simulink model "mavros_simulink_test"  (R2024b)
settings: Solver=FixedStepAuto  StartTime=0.0  StopTime=inf  FixedStep=0.01  RelTol=1e-3
undefined symbols (not defined in the file): altitude, coordinate_frame, custom_mode, custom_mode_SL_Info, latitude, longitude, min_pitch, position, start_index, type_mask, waypoints, waypoints_SL_Info, yaw
libraries: ros2lib x14, simulink_extras x1, robotcorelib x1, aerolibconvert2 x1
settings Model: Creator=hiro  LastModifiedBy=hiro

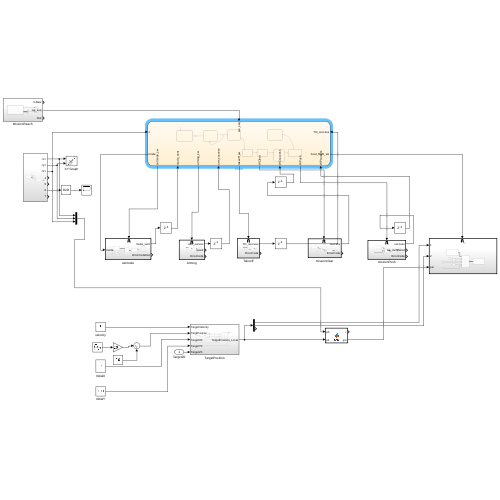
[thumbnail: Simulink's stored preview of the top-level diagram]
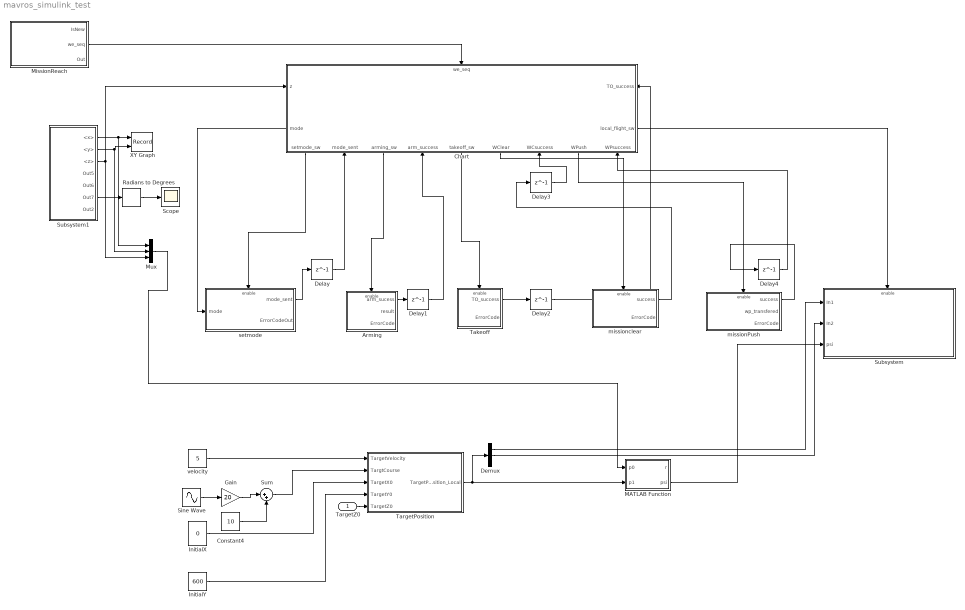
== system mavros_simulink_test ==
  TargetZ0 : Inport
  Arming : Subsystem
  Chart : Stateflow chart  TreatAsAtomicUnit=on
      settings: PortSchema="{\"entries\":[{\"content\":{\"sides\":[{\"content\":{\"connectorIds\":[\"In2\",\"Out1\"]},\"type\":\"ConnectorPlacement.EquallySpacedRectSide\",\"uuid\":\"83bdd756-f1da-4c0c-8304-adf84ef4ab4e\"},{\"content\":{\"connectorIds\":[\"In3\",\"Out2\"],\"side\":\"RIGHT\"},\"type\":\"ConnectorPlacement.EquallySpacedRectSide\",\"uuid\":\"a37bf1db-0ec9-4e4d-8590-be40530fb588\"},{\"content\":{\"connectorIds\":[\"In1\"],\"side\":\"TOP\"},\"type\":\"ConnectorPlacement.EquallySpacedRectSide\",\"uuid\":\"a8adb6fc-024d-410d-a7f4-a90207d0e0c2\"},{\"content\":{\"connectorIds\":[\"Out3\",\"In6\",\"Out4\",\"In7\",\"Out5\",\"Out6\",\"In4\",\"Out7\",\"In5\"],\"side\":\"BOTTOM\"},\"type\":\"ConnectorPlacement.EquallySpacedRectSide\",\"uuid\":\"fe5d25e7-d449-445c-b7fc-97e28e307bb9\"}]},\"type\":\"ConnectorPlacement.EquallySpacedConnector\",\"uuid\":\"da6e0aaf-ad56-47fd-8214-9fe2a8d7ed6f\"}],\"packageUris\":[\"http://schema.mathworks.com/mf0/Connector/R2020b\"],\"version\":\"1.0\"}"
  Constant4 : Constant  Value=10  SampleTime=0
  Delay{,1..4} (5 alike) : Delay  DelayLength=1  InitialCondition=0
  Demux : Demux  Outputs=3
  Gain : Gain  Gain=20
  InitialX : Constant  Value=0
  InitialY : Constant  Value=600
  MATLAB Function : MATLAB Function  TreatAsAtomicUnit=on
  MissionReach : Subsystem
  Mux : Mux  Inputs=3
  Radians to Degrees : simulink_extras/Transformations/Radians to Degrees
  Scope : Scope
  Sine Wave : Sin  Frequency=0.1  SampleTime=0
  Subsystem : Subsystem
  Subsystem1 : Subsystem
  Sum : Sum  Inputs=|++
  Takeoff : Subsystem
  TargetPosition : Subsystem
  XY Graph : Record  FileSettingsInternal="{\"entries\":[{\"content\":{\"excelSettings\":{\"content\":{},\"type\":\"Streamout.ExcelSettings\"}},\"type\":\"Streamout.FileSettingStorage\",\"uuid\":\"\"}],\"packageUris\":[\"http:\\/\\/schema.mathworks.com\\/mf0\\/streamout_blocks\\/R2020a\"],\"version\":\"1.0\"}"  Layout=[1 1]  SignalsInternal="{\"entries\":[{\"content\":{\"signals\":[{\"content\":{\"blockPath\":[],\"dimensions\":[1],\"domain\":\"\",\"lineColor\":\"#a2142f\",\"plots\":[ 1 ],\"port\":1,\"sid\":[\"\"],\"signalID\":1,\"signalName\":\"Subsystem1:1\"},\"type\":\"RecordBlkView.Signal\",\"uuid\":\"\"},{\"content\":{\"blockPath\":[],\"dimensions\":[1],\"domain\":\"\",\"lineColor\":\"#139fff\",\"plots\":[ 1 ],\"port\":2,\"sid\":[\"\"],\"signalID\":2,\"signalName\":\"Subsystem1:2\"},\"type\":\"RecordBlkView.Signal\",\"uuid\":\"\"}]},\"type\":\"RecordBlkView.InputSignals\",\"uuid\":\"\"}],\"packageUris\":[\"http:\\/\\/schema.mathworks.com\\/mf0\\/streamout_blocks\\/R2020a\"],\"version\":\"1.0\"}"  VisualizationBindings="{\"xyplotplugin\":{\"info\":[{\"series\":[{\"bindingParametersList\":[{\"parameter\":\"X-Axis\",\"signalID\":1,\"signalName\":\"Subsystem1:1\"},{\"parameter\":\"Y-Axis\",\"signalID\":2,\"signalName\":\"Subsystem1:2\"}],\"seriesID\":0}],\"subplotID\":1}]}}"  CompatibilityTag=XY
  missionPush : Subsystem
  missionclear : Subsystem
  setmode : Subsystem
  velocity : Constant  Value=5
  wires:
  Chart/2(local_flight_sw) -> Subsystem/Enable
  Subsystem1/1(<x>) -> Mux/1, XY Graph/1
  Subsystem1/2(<y>) -> Mux/2, XY Graph/2
  MATLAB Function/2(psi) -> Subsystem/3(psi)
  Subsystem1/6(Out7) -> Radians to Degrees/1
  Radians to Degrees/1 -> Scope/1
  Chart/3(setmode_sw) -> setmode/Enable
  Chart/4(arming_sw) -> Arming/Enable
  setmode/1(mode_sent) -> Delay/1
  Delay/1 -> Chart/6(mode_sent)
  Chart/1(mode) -> setmode/1(mode)
  Arming/1(arm_sucess) -> Delay1/1
  Delay1/1 -> Chart/7(arm_success)
  Chart/5(takeoff_sw) -> Takeoff/Enable
  Takeoff/1(TO_success) -> Delay2/1
  Delay2/1 -> Chart/3(TO_success)
  Subsystem1/3(<z>) -> Chart/2(z), Mux/3
  Chart/6(WClear) -> missionclear/Enable
  Chart/7(WPush) -> missionPush/Enable
  missionclear/1(success) -> Delay3/1
  missionPush/1(success) -> Delay4/1
  Delay3/1 -> Chart/4(WCsuccess)
  Delay4/1 -> Chart/5(WPsuccess)
  MissionReach/2(we_seq) -> Chart/1(we_seq)
  TargetZ0/1 -> TargetPosition/5(TargetZ0)
  TargetPosition/1(TargetPosition_Local) -> MATLAB Function/2(p1), Demux/1
  Demux/2 -> Subsystem/2(In2)
  Sine Wave/1 -> Gain/1
  Sum/1 -> TargetPosition/2(TargtCourse)
  Demux/1 -> Subsystem/1(In1)
  Constant4/1 -> Sum/2
  InitialX/1 -> TargetPosition/3(TargetX0)
  Gain/1 -> Sum/1
  InitialY/1 -> TargetPosition/4(TargetY0)
  velocity/1 -> TargetPosition/1(TargetVelocity)
  Mux/1 -> MATLAB Function/1(p0)

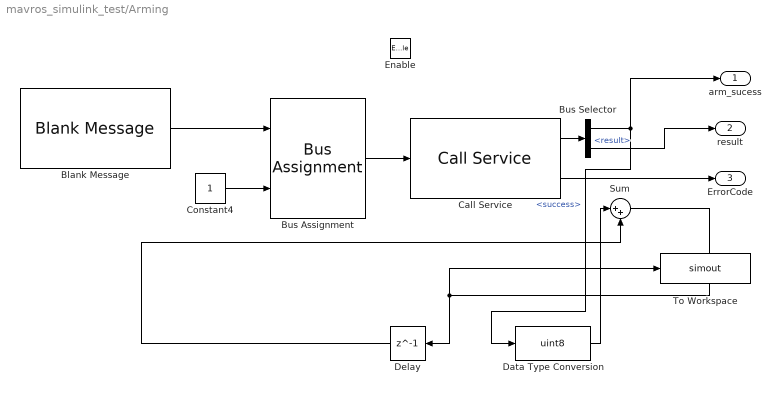
== system mavros_simulink_test/Arming ==
  Enable : EnablePort
  Blank Message : ros2lib/Blank Message  messageClass=Service Request  entityType=mavros_msgs/CommandBool  messageType=mavros_msgs/CommandBoolRequest  SampleTime=0
  Bus Assignment : BusAssignment  AssignedSignals=value
  Bus Selector : BusSelector  OutputSignals=success,result
  Call Service : ros2lib/Call Service  topicSource=Select from ROS network  service=/mavros/cmd/arming  serviceType=mavros_msgs/CommandBool  connectionTimeout=5  ShowErrorCodeOutput=on  legacyBusStruct=off  QOSHistory=Keep all  QOSDepth=1  QOSReliability=Reliable  QOSDurability=Volatile  QOSDeadline=Inf  QOSLifespan=Inf  QOSLiveliness=Automatic  QOSLeaseDuration=Inf  QOSAvoidROSNamespaceConventions=off
  Constant4 : Constant  OutDataTypeStr=boolean  SampleTime=0
  Data Type Conversion : DataTypeConversion  OutDataTypeStr=uint8  SaturateOnIntegerOverflow=off  RndMeth=Floor
  Delay : Delay  DelayLength=1  InitialCondition=0
  Sum : Sum  Inputs=|++
  To Workspace : ToWorkspace  VariableName=simout  SaveFormat=Timeseries  SampleTime=-1
  arm_sucess : Outport
  result : Outport  Port=2
  ErrorCode : Outport  Port=3
  wires:
  Call Service/2 -> ErrorCode/1
  Bus Selector/2 -> result/1  "<result>"
  Bus Selector/1 -> Data Type Conversion/1, arm_sucess/1  "<success>"
  Call Service/1 -> Bus Selector/1
  Blank Message/1 -> Bus Assignment/1
  Bus Assignment/1 -> Call Service/1
  Constant4/1 -> Bus Assignment/2
  Sum/1 -> To Workspace/1, Delay/1
  Delay/1 -> Sum/2
  Data Type Conversion/1 -> Sum/1

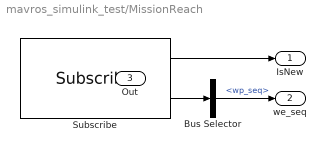
== system mavros_simulink_test/MissionReach ==
  Bus Selector : BusSelector  OutputSignals=wp_seq
  Subscribe : ros2lib/Subscribe  topicSource=Select from ROS network  topic=/mavros/mission/reached  messageType=mavros_msgs/WaypointReached  sampleTime=0  QOSHistory=Keep last  QOSDepth=1  QOSReliability=Reliable  QOSDurability=Volatile  QOSDeadline=Inf  QOSLifespan=Inf  QOSLiveliness=Automatic  QOSLeaseDuration=Inf  QOSAvoidROSNamespaceConventions=off
  IsNew : Outport
  we_seq : Outport  Port=2
  Out : Outport  Port=3
  wires:
  Subscribe/2 -> Bus Selector/1
  Subscribe/1 -> IsNew/1
  Bus Selector/1 -> we_seq/1  "<wp_seq>"

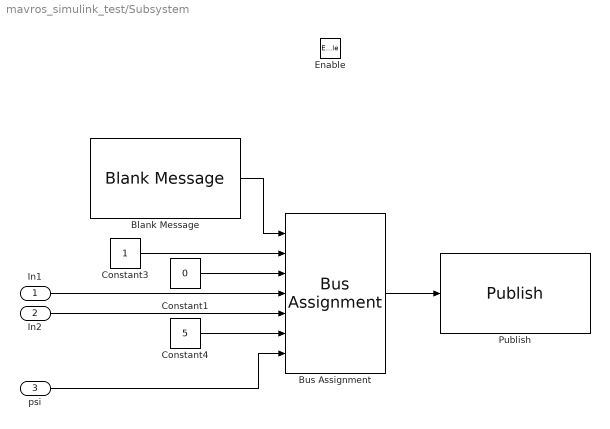
== system mavros_simulink_test/Subsystem ==
  In1 : Inport
  In2 : Inport  Port=2
  psi : Inport  Port=3
  Enable : EnablePort
  Blank Message : ros2lib/Blank Message  messageClass=Message  entityType=mavros_msgs/PositionTarget  messageType=mavros_msgs/PositionTarget  SampleTime=0
  Bus Assignment : BusAssignment  AssignedSignals=coordinate_frame,type_mask,position.x,position.y,position.z,yaw
  Constant1 : Constant  Value=0  OutDataTypeStr=uint16  SampleTime=0
  Constant3 : Constant  OutDataTypeStr=uint8  SampleTime=0
  Constant4 : Constant  Value=5  OutDataTypeStr=double  SampleTime=0
  Publish : ros2lib/Publish  topicSource=Select from ROS network  topic=/mavros/setpoint_raw/local  messageType=mavros_msgs/PositionTarget  QOSHistory=Keep last  QOSDepth=1  QOSReliability=Best effort  QOSDurability=Volatile  QOSDeadline=Inf  QOSLifespan=Inf  QOSLiveliness=Automatic  QOSLeaseDuration=Inf  QOSAvoidROSNamespaceConventions=off
  wires:
  Constant4/1 -> Bus Assignment/6
  Constant1/1 -> Bus Assignment/3
  Constant3/1 -> Bus Assignment/2
  Blank Message/1 -> Bus Assignment/1
  In1/1 -> Bus Assignment/4
  psi/1 -> Bus Assignment/7
  Bus Assignment/1 -> Publish/1
  In2/1 -> Bus Assignment/5

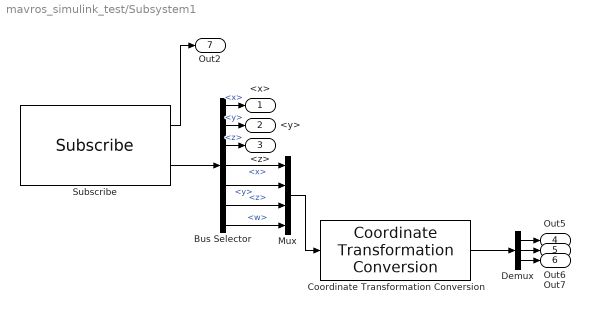
== system mavros_simulink_test/Subsystem1 ==
  Bus Selector : BusSelector  OutputSignals=pose.position.x,pose.position.y,pose.position.z,pose.orientation.x,pose.orientation.y,pose.orientation.z,pose.orientation.w
  Coordinate Transformation Conversion : robotcorelib/Coordinate Transformation Conversion  InputRepresentation=Quaternion  InputEulerSequence=ZYX  ShowTrVecInputPort=on  OutputRepresentation=Euler Angles  OutputEulerSequence=ZYX  ShowTrVecOutputPort=on  SimulateUsing=Interpreted execution
  Demux : Demux  Outputs=3
  Mux : Mux
  Subscribe : ros2lib/Subscribe  topicSource=Select from ROS network  topic=/mavros/local_position/pose  messageType=geometry_msgs/PoseStamped  sampleTime=0.01  QOSHistory=Keep last  QOSDepth=1  QOSReliability=Best effort  QOSDurability=Volatile  QOSDeadline=Inf  QOSLifespan=Inf  QOSLiveliness=Automatic  QOSLeaseDuration=Inf  QOSAvoidROSNamespaceConventions=off
  <x> : Outport
  <y> : Outport  Port=2
  <z> : Outport  Port=3
  Out5 : Outport  Port=4
  Out6 : Outport  Port=5
  Out7 : Outport  Port=6
  Out2 : Outport  Port=7
  wires:
  Demux/3 -> Out7/1
  Subscribe/2 -> Bus Selector/1
  Bus Selector/7 -> Mux/4  "<w>"
  Bus Selector/2 -> <y>/1  "<y>"
  Bus Selector/4 -> Mux/1  "<x>"
  Coordinate Transformation Conversion/1 -> Demux/1
  Bus Selector/6 -> Mux/3  "<z>"
  Bus Selector/1 -> <x>/1  "<x>"
  Bus Selector/5 -> Mux/2  "<y>"
  Demux/1 -> Out5/1
  Demux/2 -> Out6/1
  Bus Selector/3 -> <z>/1  "<z>"
  Mux/1 -> Coordinate Transformation Conversion/1
  Subscribe/1 -> Out2/1

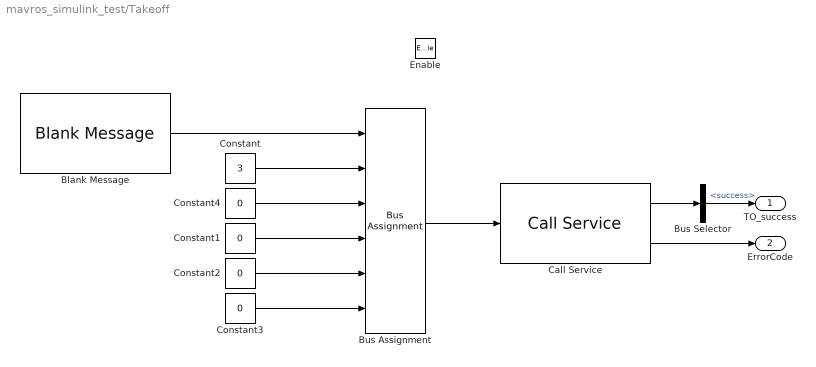
== system mavros_simulink_test/Takeoff ==
  Enable : EnablePort
  Blank Message : ros2lib/Blank Message  messageClass=Service Request  entityType=mavros_msgs/CommandTOL  messageType=mavros_msgs/CommandTOLRequest  SampleTime=0
  Bus Assignment : BusAssignment  AssignedSignals=altitude,latitude,longitude,min_pitch,yaw
  Bus Selector : BusSelector  OutputSignals=success
  Call Service : ros2lib/Call Service  topicSource=Select from ROS network  service=/mavros/cmd/takeoff  serviceType=mavros_msgs/CommandTOL  connectionTimeout=5  ShowErrorCodeOutput=on  legacyBusStruct=off  QOSHistory=Keep last  QOSDepth=1  QOSReliability=Reliable  QOSDurability=Volatile  QOSDeadline=Inf  QOSLifespan=Inf  QOSLiveliness=Automatic  QOSLeaseDuration=Inf  QOSAvoidROSNamespaceConventions=off
  Constant : Constant  Value=3  OutDataTypeStr=single  SampleTime=0
  Constant{1..4} (4 alike) : Constant  Value=0  OutDataTypeStr=single  SampleTime=0
  TO_success : Outport
  ErrorCode : Outport  Port=2
  wires:
  Bus Assignment/1 -> Call Service/1
  Call Service/2 -> ErrorCode/1
  Constant4/1 -> Bus Assignment/3
  Blank Message/1 -> Bus Assignment/1
  Constant/1 -> Bus Assignment/2
  Constant1/1 -> Bus Assignment/4
  Constant2/1 -> Bus Assignment/5
  Constant3/1 -> Bus Assignment/6
  Call Service/1 -> Bus Selector/1
  Bus Selector/1 -> TO_success/1  "<success>"

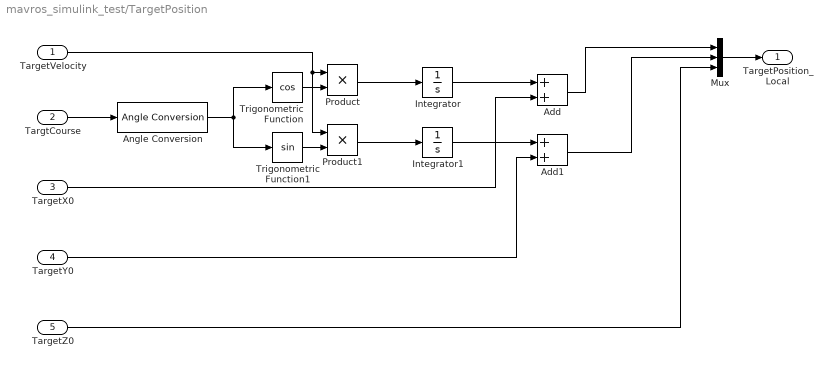
== system mavros_simulink_test/TargetPosition ==
  TargetVelocity : Inport
  TargtCourse : Inport  Port=2
  TargetX0 : Inport  Port=3
  TargetY0 : Inport  Port=4
  TargetZ0 : Inport  Port=5
  Add : Sum
  Add1 : Sum
  Angle Conversion : aerolibconvert2/Angle Conversion  IU=deg  OU=rad
  Integrator : Integrator
  Integrator1 : Integrator
  Mux : Mux  Inputs=3
  Product : Product
  Product1 : Product
  Trigonometric Function : Trigonometry  Operator=cos
  Trigonometric Function1 : Trigonometry
  TargetPosition_Local : Outport
  wires:
  Mux/1 -> TargetPosition_Local/1
  TargetZ0/1 -> Mux/3
  TargetVelocity/1 -> Product/1, Product1/1
  Add/1 -> Mux/1
  Trigonometric Function1/1 -> Product1/2
  Product/1 -> Integrator/1
  Trigonometric Function/1 -> Product/2
  TargetX0/1 -> Add/2
  Angle Conversion/1 -> Trigonometric Function/1, Trigonometric Function1/1
  Add1/1 -> Mux/2
  Integrator/1 -> Add/1
  Integrator1/1 -> Add1/1
  TargtCourse/1 -> Angle Conversion/1
  Product1/1 -> Integrator1/1
  TargetY0/1 -> Add1/2

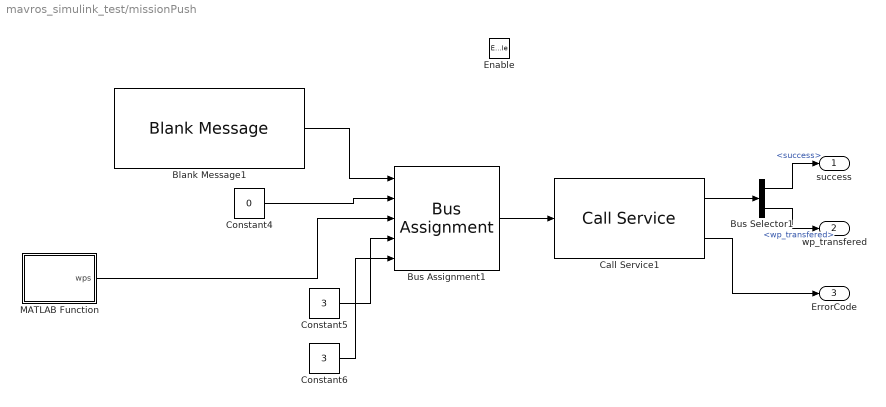
== system mavros_simulink_test/missionPush ==
  Enable : EnablePort
  Blank Message1 : ros2lib/Blank Message  messageClass=Service Request  entityType=mavros_msgs/WaypointPush  messageType=mavros_msgs/WaypointPushRequest  SampleTime=0
  Bus Assignment1 : BusAssignment  AssignedSignals=start_index,waypoints,waypoints_SL_Info.CurrentLength,waypoints_SL_Info.ReceivedLength
  Bus Selector1 : BusSelector  OutputSignals=success,wp_transfered
  Call Service1 : ros2lib/Call Service  topicSource=Select from ROS network  service=/mavros/mission/push  serviceType=mavros_msgs/WaypointPush  connectionTimeout=5  ShowErrorCodeOutput=on  legacyBusStruct=off  QOSHistory=Keep last  QOSDepth=1  QOSReliability=Reliable  QOSDurability=Volatile  QOSDeadline=Inf  QOSLifespan=Inf  QOSLiveliness=Automatic  QOSLeaseDuration=Inf  QOSAvoidROSNamespaceConventions=off
  Constant4 : Constant  Value=0  OutDataTypeStr=uint16  SampleTime=0
  Constant5 : Constant  Value=3  OutDataTypeStr=uint32  SampleTime=0
  Constant6 : Constant  Value=3  OutDataTypeStr=uint32  SampleTime=0
  MATLAB Function : MATLAB Function  TreatAsAtomicUnit=on
  success : Outport
  wp_transfered : Outport  Port=2
  ErrorCode : Outport  Port=3
  wires:
  Bus Selector1/1 -> success/1  "<success>"
  Bus Assignment1/1 -> Call Service1/1
  Constant4/1 -> Bus Assignment1/2
  Bus Selector1/2 -> wp_transfered/1  "<wp_transfered>"
  Blank Message1/1 -> Bus Assignment1/1
  MATLAB Function/1(wps) -> Bus Assignment1/3
  Constant6/1 -> Bus Assignment1/5
  Constant5/1 -> Bus Assignment1/4
  Call Service1/1 -> Bus Selector1/1
  Call Service1/2 -> ErrorCode/1

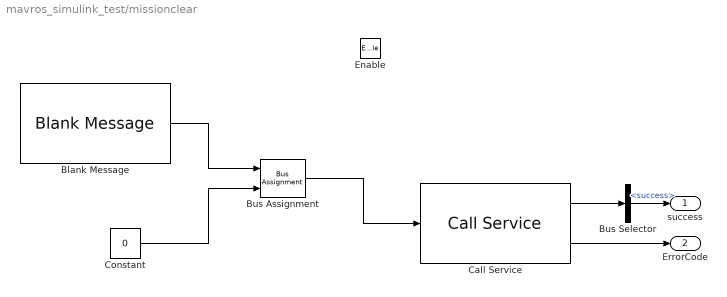
== system mavros_simulink_test/missionclear ==
  Enable : EnablePort
  Blank Message : ros2lib/Blank Message  messageClass=Service Request  entityType=mavros_msgs/WaypointClear  messageType=mavros_msgs/WaypointClearRequest  SampleTime=0
  Bus Assignment : BusAssignment  AssignedSignals=SL_DummyData
  Bus Selector : BusSelector  OutputSignals=success
  Call Service : ros2lib/Call Service  topicSource=Select from ROS network  service=/mavros/mission/clear  serviceType=mavros_msgs/WaypointClear  connectionTimeout=5  ShowErrorCodeOutput=on  legacyBusStruct=off  QOSHistory=Keep last  QOSDepth=1  QOSReliability=Reliable  QOSDurability=Volatile  QOSDeadline=Inf  QOSLifespan=Inf  QOSLiveliness=Automatic  QOSLeaseDuration=Inf  QOSAvoidROSNamespaceConventions=off
  Constant : Constant  Value=0  OutDataTypeStr=boolean  SampleTime=0
  success : Outport
  ErrorCode : Outport  Port=2
  wires:
  Bus Assignment/1 -> Call Service/1
  Blank Message/1 -> Bus Assignment/1
  Bus Selector/1 -> success/1  "<success>"
  Call Service/2 -> ErrorCode/1
  Call Service/1 -> Bus Selector/1
  Constant/1 -> Bus Assignment/2

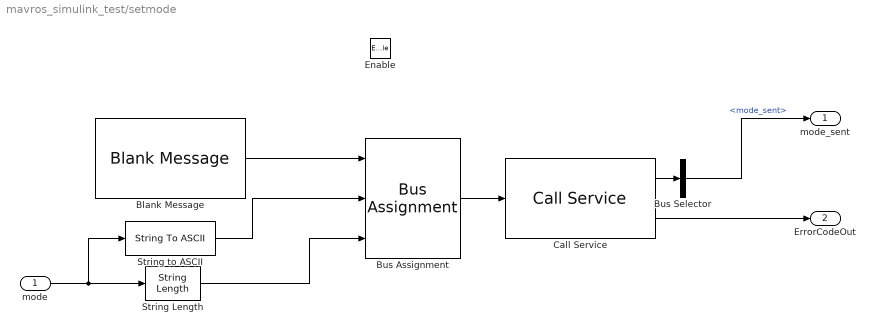
== system mavros_simulink_test/setmode ==
  mode : Inport
  Enable : EnablePort
  Blank Message : ros2lib/Blank Message  messageClass=Service Request  entityType=mavros_msgs/SetMode  messageType=mavros_msgs/SetModeRequest  SampleTime=0
  Bus Assignment : BusAssignment  AssignedSignals=custom_mode,custom_mode_SL_Info.CurrentLength
  Bus Selector : BusSelector  OutputSignals=mode_sent
  Call Service : ros2lib/Call Service  topicSource=Select from ROS network  service=/mavros/set_mode  serviceType=mavros_msgs/SetMode  connectionTimeout=5  ShowErrorCodeOutput=on  legacyBusStruct=off  QOSHistory=Keep all  QOSDepth=1  QOSReliability=Reliable  QOSDurability=Volatile  QOSDeadline=Inf  QOSLifespan=Inf  QOSLiveliness=Automatic  QOSLeaseDuration=Inf  QOSAvoidROSNamespaceConventions=off
  String Length : StringLength
  String to ASCII : StringToASCII  OutputVectorSize=128
  mode_sent : Outport
  ErrorCodeOut : Outport  Port=2
  wires:
  Bus Assignment/1 -> Call Service/1
  Call Service/1 -> Bus Selector/1
  String Length/1 -> Bus Assignment/3
  Blank Message/1 -> Bus Assignment/1
  Call Service/2 -> ErrorCodeOut/1
  mode/1 -> String Length/1, String to ASCII/1
  String to ASCII/1 -> Bus Assignment/2
  Bus Selector/1 -> mode_sent/1  "<mode_sent>"

== matlab function mavros_simulink_test/MATLAB Function ==
  data: p0 input; r output; p1 input; psi output
function [r,psi] = fcn(p0,p1)

r=sqrt((p0(1)-p1(1))^2+(p0(2)-p1(2))^2+(p0(3)-p1(3))^2);
psi = single(atan2(p1(2)-p0(2),p1(1)-p0(1)));

== matlab function mavros_simulink_test/missionPush/MATLAB Function ==
  data: wps output Bus: SL_Bus_mavros_msgs_Waypoint size=16
function wps = fcn()


wp0.frame = uint8(3);  % MAV_FRAME_GLOBAL_REL_ALT
wp0.command = uint16(16);  % MAV_CMD_NAV_WAYPOINT
wp0.is_current = true;
wp0.autocontinue = true;
wp0.param1 = single(0);
wp0.param2 = single(0);
wp0.param3 = single(0);
wp0.param4 = single(0);
wp0.x_lat = double(32.698307);  % 緯度
wp0.y_long = double(129.783437); % 経度
wp0.z_alt = double(10);         % 高度[m]


wp1.frame = uint8(3);  % MAV_FRAME_GLOBAL_REL_ALT
wp1.command = uint16(16);  % MAV_CMD_NAV_WAYPOINT
wp1.is_current = false;
wp1.autocontinue = true;
wp1.param1 = single(0);
wp1.param2 = single(0);
wp1.param3 = single(0);
wp1.param4 = single(0);
wp1.x_lat = double(32.697292);  % 緯度
wp1.y_long = double(129.784437); % 経度
wp1.z_alt = double(10);         % 高度[m]

wp2.frame = uint8(3);  % MAV_FRAME_GLOBAL_REL_ALT
wp2.command = uint16(16);  % MAV_CMD_NAV_WAYPOINT
wp2.is_current = false;
wp2.autocontinue = true;
wp2.param1 = single(0);
wp2.param2 = single(0);
wp2.param3 = single(0);
wp2.param4 = single(0);
wp2.x_lat = double(32.698020);  % 緯度
wp2.y_long = double(129.785450); % 経度
wp2.z_alt = double(10);         % 高度[m]


wp3.frame = uint8(0);  % MAV_FRAME_GLOBAL_REL_ALT
wp3.command = uint16(0);  % MAV_CMD_NAV_WAYPOINT
wp3.is_current = false;
wp3.autocontinue = false;
wp3.param1 = single(0);
wp3.param2 = single(0);
wp3.param3 = single(0);
wp3.param4 = single(0);
wp3.x_lat = double(0);  % 緯度
wp3.y_long = double(0); % 経度
wp3.z_alt = double(0);         % 高度[m]

wp4=wp3;
wp5=wp3;
wp6=wp3;
wp7=wp3;
wp8=wp3;
wp9=wp3;
wp10=wp3;
wp11=wp3;
wp12=wp3;
wp13=wp3;
wp14=wp3;
wp15=wp3;

wps = [wp0;wp1;wp2;wp3;wp4;wp5;wp6;wp7;wp8;wp9;wp10;wp11;wp12;wp13;wp14;wp15];

== stateflow chart mavros_simulink_test/Chart ==
  state Takeoff
    entry:
    takeoff_sw=1;
    arming_sw=0;
  state Flight
    entry:
    local_flight_sw=1;
    setmode_sw=0;
  state Start
    entry:
    setmode_sw=1;
    mode="GUIDED";
  state Arming
    entry:
    arming_sw=1;
    setmode_sw=0;
  state WaypointClear
    entry:
    WClear=1;
    takeoff_sw=0;
  state WaypointPush
    entry:
    WPush=1;
    WClear=0;
  state Auto
    entry:
    WPush=0;
    setmode_sw=1;
    mode="AUTO"
  state start_persuit
    entry:
    setmode_sw=1
    mode="GUIDED";
  (default) -> Start
  (junction 42) -> Takeoff [order 1] : [arm_success==1]
  Arming -> (junction 42) : after(1,sec)
  start_persuit -> Flight : [mode_sent==1]
  (junction 42) -> Arming [order 2] : [arm_success==0]
  Start -> (junction 40) : after(1,sec)
  (junction 40) -> Arming : [[mode_sent==1]]
  Takeoff -> WaypointClear : [z>=2]
  WaypointPush -> Auto : [WPsuccess==1]
  WaypointClear -> WaypointPush : [WCsuccess==1]
  Auto -> start_persuit : [we_seq==2]
  data: we_seq input; z input; TO_success input; WCsuccess input; WPsuccess input; mode output; local_flight_sw output; setmode_sw output; arming_sw output; mode_sent input; arm_success input; takeoff_sw output; WClear output; WPush output
